simulink model "test_beta_estimator"  (R2017a)
settings: Solver=VariableStepAuto  StartTime=0.0  StopTime=10  FixedStep=SIM_Tsolver  MaxStep=1e-3  RelTol=1e-4  AbsTol=1e-4
values from neighbouring files (symbols this model uses):
  ROS_clockPublishingPeriod = 1e-3    (= 0.001)    [test_beta_estimator_init.m]
  ROS_measurementPublishingPeriod = 1e-2    (= 0.01)    [test_beta_estimator_init.m]
  SIM_Tsolver = 1e-4    (= 0.0001)    [test_beta_estimator_init.m]
undefined symbols (not defined in the file or in its folder): Clock_, Theta, X, Y
libraries: robotlib x5
settings Model: SimulationMode=accelerator  ExtModeTrigDuration=100  Creator=Alessandro  LastModifiedBy=bascetta
settings SolverCC: MaxConsecutiveMinStep=10  ZeroCrossControl=DisableAll
settings DataIOCC: SaveFormat=StructureWithTime  SaveOutput=off  SaveTime=off  StateSaveName=tmp_raccel_xout  TimeSaveName=t_out  SignalLoggingName=SDO_logsout
settings OptimizationCC: EfficientMapNaN2IntZero=off  LifeSpan=inf
settings DebuggingCC: SFUnexpectedBacktrackingDiag=warning  SFNoUnconditionalDefaultTransitionDiag=warning  SFExecutionAtInitializationDiag=none
settings HardwareCC: ProdBitPerPointer=32  ProdBitPerSizeT=32  ProdBitPerPtrDiffT=32  ProdLargestAtomicFloat=None  ProdIntDivRoundTo=Undefined  ProdEndianess=Unspecified  ProdWordSize=32  ProdHWDeviceType=32-bit Generic  TargetBitPerLong=64  TargetBitPerPointer=64  TargetBitPerSizeT=64  TargetBitPerPtrDiffT=64  TargetLongLongMode=on  TargetIntDivRoundTo=Zero  TargetEndianess=LittleEndian  TargetWordSize=64  TargetHWDeviceType=MATLAB Host  ProdEqTarget=off
settings ModelReferenceCC: PropagateSignalLabelsOutOfModel=off
settings CodeAppCC: MaxIdLength=128
settings GRTTargetCC: TargetLangStandard=C89/C90 (ANSI)  GeneratePreprocessorConditionals=Disable all  CombineOutputUpdateFcns=off  GRTInterface=on
settings ConfigComp: CovMetricSettings=dw  CovHtmlReporting=on  CovSaveCumulativeToWorkspaceVar=on  CovSaveSingleToWorkspaceVar=on  CovExternalEMLEnable=off

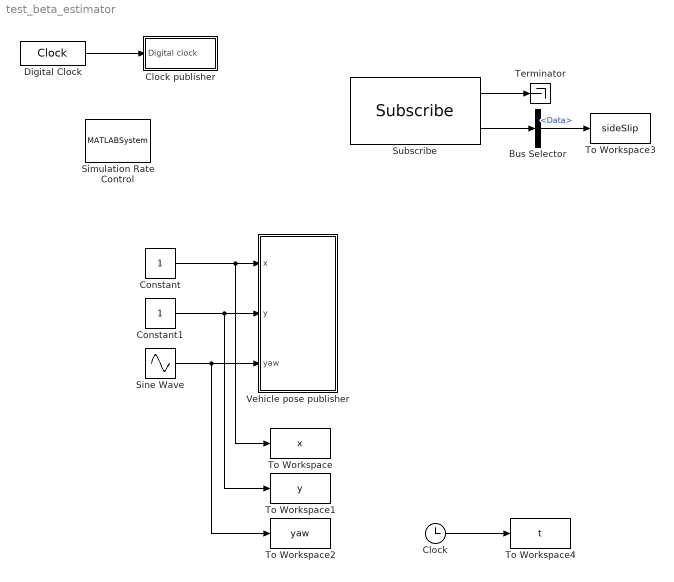
== system test_beta_estimator ==
  Bus Selector : BusSelector  OutputSignals=Data
  Clock : Clock
  Clock publisher : Subsystem
  Constant : Constant
  Constant1 : Constant
  Digital Clock : DigitalClock  SampleTime=SIM_Tsolver
  Simulation Rate Control : MATLABSystem  System=ExampleHelperSimulationRateControl  SampleTime=SIM_Tsolver
      mask Type: ExampleHelperSimulationRateControl
      mask Display: disp('Rate Control');
  Sine Wave : Sin  SampleTime=0
  Subscribe : robotlib/Subscribe  SourceLibraryInfo=This block requires Robotics System Toolbox  topicSource=Select from ROS network  topic=/vehicleSideslip  messageType=std_msgs/Float64  sampleTime=-1  messageQueueLength=1
      settings: SourceProductBaseCode=RO
  Terminator : Terminator
  To Workspace : ToWorkspace  VariableName=x  SampleTime=-1
      settings: Save2DSignal=2-D array (concatenate along first dimension)
  To Workspace1 : ToWorkspace  VariableName=y  SampleTime=-1
      settings: Save2DSignal=2-D array (concatenate along first dimension)
  To Workspace2 : ToWorkspace  VariableName=yaw  SampleTime=-1
      settings: Save2DSignal=2-D array (concatenate along first dimension)
  To Workspace3 : ToWorkspace  VariableName=sideSlip  SampleTime=-1
      settings: Save2DSignal=2-D array (concatenate along first dimension)
  To Workspace4 : ToWorkspace  VariableName=t  SampleTime=-1
      settings: Save2DSignal=2-D array (concatenate along first dimension)
  Vehicle pose publisher : Subsystem
  wires:
  Digital Clock/1 -> Clock publisher/1(Digital clock)
  Sine Wave/1 -> To Workspace2/1, Vehicle pose publisher/3(yaw)
  Constant1/1 -> To Workspace1/1, Vehicle pose publisher/2(y)
  Constant/1 -> To Workspace/1, Vehicle pose publisher/1(x)
  Subscribe/1 -> Terminator/1
  Clock/1 -> To Workspace4/1
  Subscribe/2 -> Bus Selector/1
  Bus Selector/1 -> To Workspace3/1  "<Data>"

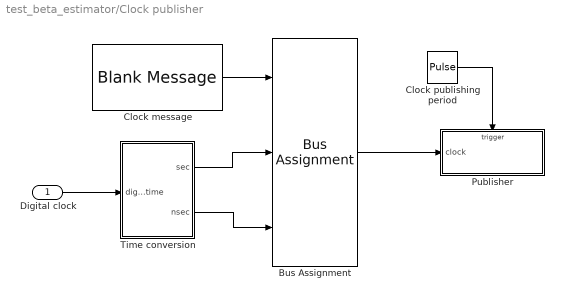
== system test_beta_estimator/Clock publisher ==
  Digital clock : Inport
  Bus Assignment : BusAssignment  DialogController=Simulink.DDGSource_BusAssignment  AssignedSignals=Clock_.Sec,Clock_.Nsec
  Clock message : robotlib/Blank Message  SourceLibraryInfo=This block requires Robotics System Toolbox  messageType=rosgraph_msgs/Clock  SampleTime=inf
      settings: SourceProductBaseCode=RO
  Clock publishing period : DiscretePulseGenerator  PulseType=Time based  Period=ROS_clockPublishingPeriod  PulseWidth=50
  Publisher : Subsystem  TreatAsAtomicUnit=on
  Time conversion : MATLAB Function  TreatAsAtomicUnit=on
  wires:
  Clock message/1 -> Bus Assignment/1
  Bus Assignment/1 -> Publisher/1(clock)
  Time conversion/1(sec) -> Bus Assignment/2
  Time conversion/2(nsec) -> Bus Assignment/3
  Digital clock/1 -> Time conversion/1(digital_time)
  Clock publishing period/1 -> Publisher/Trigger

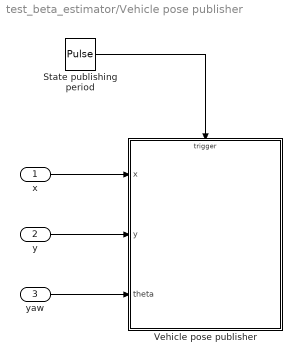
== system test_beta_estimator/Vehicle pose publisher ==
  x : Inport
  y : Inport  Port=2
  yaw : Inport  Port=3
  State publishing period : DiscretePulseGenerator  PulseType=Time based  Period=ROS_measurementPublishingPeriod  PulseWidth=50
  Vehicle pose publisher : Subsystem  TreatAsAtomicUnit=on
  wires:
  State publishing period/1 -> Vehicle pose publisher/Trigger
  x/1 -> Vehicle pose publisher/1(x)
  y/1 -> Vehicle pose publisher/2(y)
  yaw/1 -> Vehicle pose publisher/3(theta)

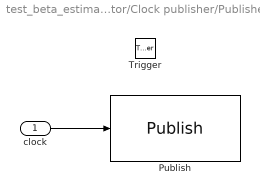
== system test_beta_estimator/Clock publisher/Publisher ==
  clock : Inport
  Trigger : TriggerPort  VariantControl=Variant
  Publish : robotlib/Publish  SourceLibraryInfo=This block requires Robotics System Toolbox  topicSource=Specify your own  topic=/clock  messageType=rosgraph_msgs/Clock  messageQueueLength=1
      settings: SourceProductBaseCode=RO
  wires:
  clock/1 -> Publish/1

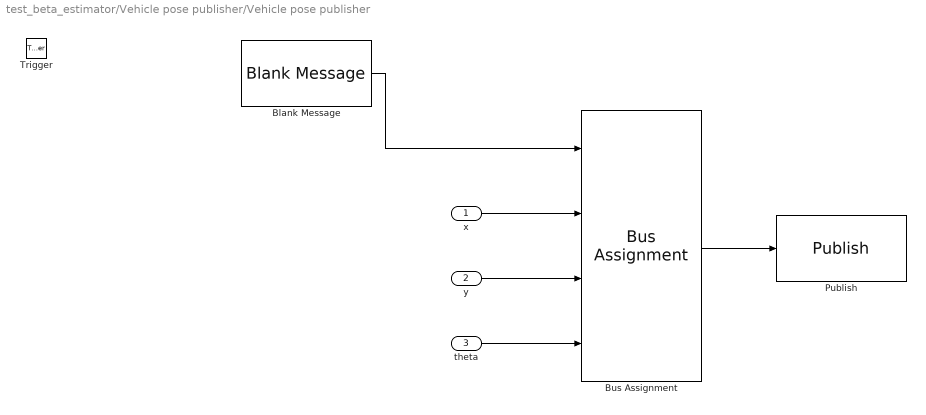
== system test_beta_estimator/Vehicle pose publisher/Vehicle pose publisher ==
  x : Inport
  y : Inport  Port=2
  theta : Inport  Port=3
  Trigger : TriggerPort  VariantControl=Variant
  Blank Message : robotlib/Blank Message  SourceLibraryInfo=This block requires Robotics System Toolbox  messageType=geometry_msgs/Pose2D  SampleTime=inf
      settings: SourceProductBaseCode=RO
  Bus Assignment : BusAssignment  DialogController=Simulink.DDGSource_BusAssignment  AssignedSignals=X,Y,Theta
  Publish : robotlib/Publish  SourceLibraryInfo=This block requires Robotics System Toolbox  topicSource=Select from ROS network  topic=/vehiclePose  messageType=geometry_msgs/Pose2D  messageQueueLength=1
      settings: SourceProductBaseCode=RO
  wires:
  Blank Message/1 -> Bus Assignment/1
  Bus Assignment/1 -> Publish/1
  theta/1 -> Bus Assignment/4
  y/1 -> Bus Assignment/3
  x/1 -> Bus Assignment/2

== matlab function test_beta_estimator/Clock publisher/Time conversion ==
  data: digital_time input; sec output; nsec output
function [sec,nsec] = time2rosclock(digital_time)

sec = floor(digital_time);
nsec = round((digital_time-sec)*1.0e+9);
